simulink model "Helicopter_DT_sol"  (R2023b)
settings: Solver=ode3  StartTime=0.0  StopTime=20  FixedStep=0.01  RelTol=1e-3
undefined symbols (not defined in the file): A, B, Kd, Nd_bar, Ts
libraries: simulink_extras x3
settings Model: Creator=jerome  LastModifiedBy=jerome
settings ModelReferenceCC: EnableRefExpFcnMdlSchedulingChecks=on

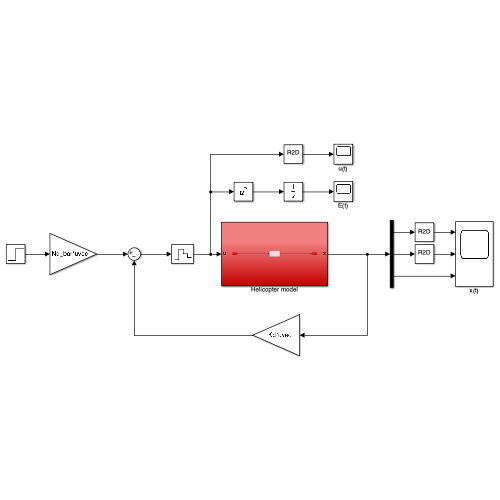
[thumbnail: Simulink's stored preview of the top-level diagram]
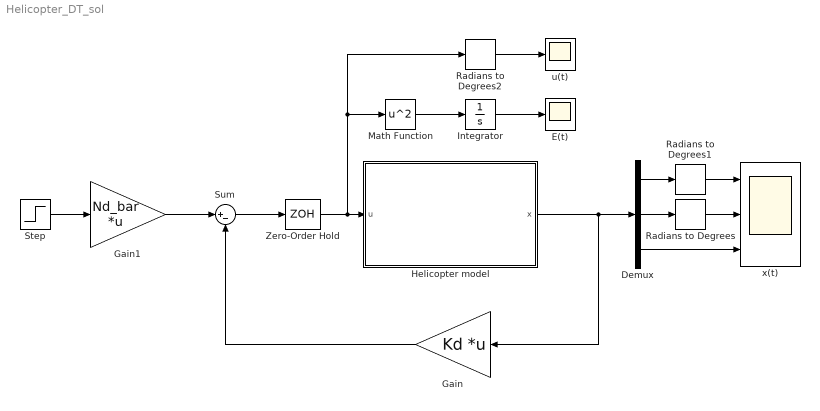
== system Helicopter_DT_sol ==
  Demux : Demux  Outputs=3
  E(t) : Scope
  Gain : Gain  Gain=Kd  Multiplication=Matrix(K*u) (u vector)
  Gain1 : Gain  Gain=Nd_bar  Multiplication=Matrix(K*u) (u vector)
  Helicopter model : Subsystem
  Integrator : Integrator
  Math Function : Math  Operator=square
  Radians to Degrees : simulink_extras/Transformations/Radians to Degrees
  Radians to Degrees1 : simulink_extras/Transformations/Radians to Degrees
  Radians to Degrees2 : simulink_extras/Transformations/Radians to Degrees
  Step : Step  After=10  SampleTime=0
  Sum : Sum  Inputs=|+-
  Zero-Order Hold : ZeroOrderHold  SampleTime=10*Ts
  u(t) : Scope
  x(t) : Scope  NumInputPorts=3
  wires:
  Helicopter model/1(x) -> Gain/1, Demux/1
  Sum/1 -> Zero-Order Hold/1
  Gain/1 -> Sum/2
  Step/1 -> Gain1/1
  Integrator/1 -> E(t)/1
  Math Function/1 -> Integrator/1
  Demux/1 -> Radians to Degrees1/1
  Demux/2 -> Radians to Degrees/1
  Demux/3 -> x(t)/3
  Radians to Degrees/1 -> x(t)/2
  Radians to Degrees1/1 -> x(t)/1
  Radians to Degrees2/1 -> u(t)/1
  Zero-Order Hold/1 -> Helicopter model/1(u), Math Function/1, Radians to Degrees2/1
  Gain1/1 -> Sum/1

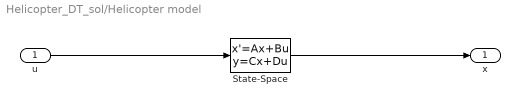
== system Helicopter_DT_sol/Helicopter model ==
  u : Inport
  State-Space : StateSpace  A=A  B=B  C=eye(3)  D=zeros(3,1)  InitialCondition=[0;0;0]
  x : Outport
  wires:
  u/1 -> State-Space/1
  State-Space/1 -> x/1
